simulink model "biplex_unscr_tail_plan"  (Simulink 7.6)
settings: Solver=ode45  StartTime=0.0  StopTime=10.0  RelTol=1e-3
libraries: xbsIndex_r4 x206, monroe_library x3
(part 1 of 2)
settings Model: Creator=monroe  LastModifiedBy=monroe

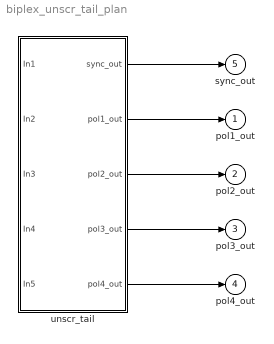
== system biplex_unscr_tail_plan ==
  unscr_tail : Subsystem  mask{FFTSize=5, input_bit_width=18, bram_latency=3, reorder_din_latency=1}
      mask prompts: FFTSize "FFT Size"; input_bit_width "Input Bit Width"; bram_latency "BRAM Latency"; reorder_din_latency "Reorder DIN Latency"
  pol1_out : Outport
  pol2_out : Outport  Port=2
  pol3_out : Outport  Port=3
  pol4_out : Outport  Port=4
  sync_out : Outport  Port=5
  wires:
  unscr_tail/5(pol4_out) -> pol4_out/1
  unscr_tail/4(pol3_out) -> pol3_out/1
  unscr_tail/3(pol2_out) -> pol2_out/1
  unscr_tail/2(pol1_out) -> pol1_out/1
  unscr_tail/1(sync_out) -> sync_out/1

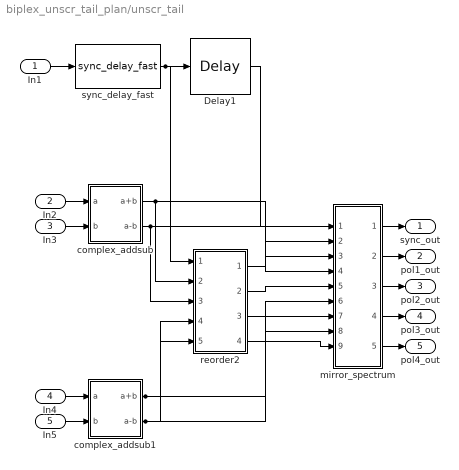
== system biplex_unscr_tail_plan/unscr_tail ==
  In1 : Inport
  In2 : Inport  Port=2
  In3 : Inport  Port=3
  In4 : Inport  Port=4
  In5 : Inport  Port=5
  Delay1 : xbsIndex_r4/Delay  en=off  latency=bram_latency + reorder_din_latency  dbl_ovrd=off  reg_retiming=off  block_type=delay
  complex_addsub : Subsystem
  complex_addsub1 : Subsystem
  mirror_spectrum : Subsystem
  reorder2 : Subsystem
  sync_delay_fast : monroe_library/sync_delay_fast  SystemSampleTime=-1  delay_len=2^(FFTSize-1) + 2
  sync_out : Outport
  pol1_out : Outport  Port=2
  pol2_out : Outport  Port=3
  pol3_out : Outport  Port=4
  pol4_out : Outport  Port=5
  wires:
  complex_addsub/2(a-b) -> reorder2/3(din1), mirror_spectrum/4(din1)
  complex_addsub/1(a+b) -> reorder2/2(din0), mirror_spectrum/2(din0)
  Delay1/1 -> mirror_spectrum/1(sync)
  reorder2/1(dout0) -> mirror_spectrum/3(reo_in0)
  reorder2/2(dout1) -> mirror_spectrum/5(reo_in1)
  reorder2/3(dout2) -> mirror_spectrum/7(reo_in2)
  reorder2/4(dout3) -> mirror_spectrum/9(reo_in3)
  complex_addsub1/2(a-b) -> mirror_spectrum/8(din3), reorder2/5(din3)
  complex_addsub1/1(a+b) -> mirror_spectrum/6(din2), reorder2/4(din2)
  sync_delay_fast/1 -> Delay1/1, reorder2/1(sync)
  In1/1 -> sync_delay_fast/1
  In2/1 -> complex_addsub/1(a)
  In3/1 -> complex_addsub/2(b)
  mirror_spectrum/1(sync_out) -> sync_out/1
  mirror_spectrum/2(dout0) -> pol1_out/1
  mirror_spectrum/3(dout1) -> pol2_out/1
  mirror_spectrum/4(dout2) -> pol3_out/1
  mirror_spectrum/5(dout3) -> pol4_out/1
  In4/1 -> complex_addsub1/1(a)
  In5/1 -> complex_addsub1/2(b)

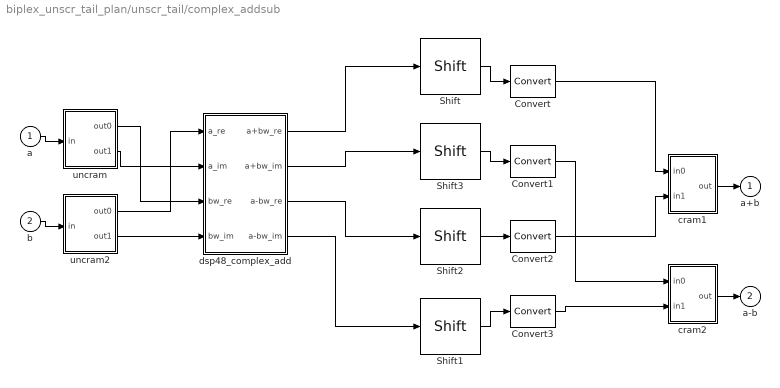
== system biplex_unscr_tail_plan/unscr_tail/complex_addsub ==
  a : Inport
  b : Inport  Port=2
  Convert{,1..3} (4 alike) : xbsIndex_r4/Convert  arith_type="Signed  (2's comp)"  n_bits=input_bit_width  bin_pt=input_bit_width-1  quantization=Truncate  overflow=Wrap  en=off  latency=0  dbl_ovrd=off  pipeline=off  block_type=convert
  Shift{,1..3} (4 alike) : xbsIndex_r4/Shift  shift_dir=Right  shift_bits=1  en=off  latency=0  precision=Full  arith_type="Signed  (2's comp)"  n_bits=8  bin_pt=2  quantization=Truncate  overflow=Wrap  dbl_ovrd=off  block_type=shift
  cram1 : Subsystem
  cram2 : Subsystem
  dsp48_complex_add : Subsystem
  uncram : Subsystem
  uncram2 : Subsystem
  a+b : Outport
  a-b : Outport  Port=2
  wires:
  a/1 -> uncram/1(in)
  b/1 -> uncram2/1(in)
  Convert/1 -> cram1/1(in0)
  Convert2/1 -> cram1/2(in1)
  cram1/1(out) -> a+b/1
  Convert1/1 -> cram2/1(in0)
  Convert3/1 -> cram2/2(in1)
  cram2/1(out) -> a-b/1
  uncram2/1(out0) -> dsp48_complex_add/1(a_re)
  uncram/2(out1) -> dsp48_complex_add/2(a_im)
  uncram/1(out0) -> dsp48_complex_add/3(bw_re)
  uncram2/2(out1) -> dsp48_complex_add/4(bw_im)
  dsp48_complex_add/1(a+bw_re) -> Shift/1
  dsp48_complex_add/2(a+bw_im) -> Shift3/1
  dsp48_complex_add/3(a-bw_re) -> Shift2/1
  dsp48_complex_add/4(a-bw_im) -> Shift1/1
  Shift1/1 -> Convert3/1
  Shift2/1 -> Convert2/1
  Shift3/1 -> Convert1/1
  Shift/1 -> Convert/1

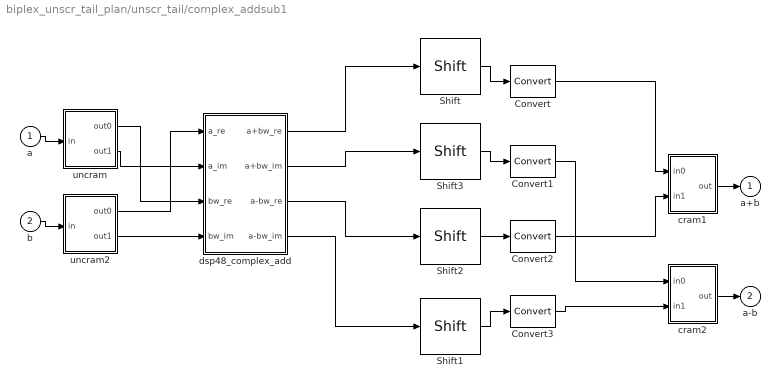
== system biplex_unscr_tail_plan/unscr_tail/complex_addsub1 ==
  a : Inport
  b : Inport  Port=2
  Convert{,1..3} (4 alike) : xbsIndex_r4/Convert  arith_type="Signed  (2's comp)"  n_bits=input_bit_width  bin_pt=input_bit_width-1  quantization=Truncate  overflow=Wrap  en=off  latency=0  dbl_ovrd=off  pipeline=off  block_type=convert
  Shift{,1..3} (4 alike) : xbsIndex_r4/Shift  shift_dir=Right  shift_bits=1  en=off  latency=0  precision=Full  arith_type="Signed  (2's comp)"  n_bits=8  bin_pt=2  quantization=Truncate  overflow=Wrap  dbl_ovrd=off  block_type=shift
  cram1 : Subsystem
  cram2 : Subsystem
  dsp48_complex_add : Subsystem
  uncram : Subsystem
  uncram2 : Subsystem
  a+b : Outport
  a-b : Outport  Port=2
  wires:
  Shift/1 -> Convert/1
  Shift3/1 -> Convert1/1
  Shift2/1 -> Convert2/1
  Shift1/1 -> Convert3/1
  dsp48_complex_add/4(a-bw_im) -> Shift1/1
  dsp48_complex_add/3(a-bw_re) -> Shift2/1
  dsp48_complex_add/2(a+bw_im) -> Shift3/1
  dsp48_complex_add/1(a+bw_re) -> Shift/1
  uncram2/2(out1) -> dsp48_complex_add/4(bw_im)
  uncram/1(out0) -> dsp48_complex_add/3(bw_re)
  uncram/2(out1) -> dsp48_complex_add/2(a_im)
  uncram2/1(out0) -> dsp48_complex_add/1(a_re)
  cram2/1(out) -> a-b/1
  Convert3/1 -> cram2/2(in1)
  Convert1/1 -> cram2/1(in0)
  cram1/1(out) -> a+b/1
  Convert2/1 -> cram1/2(in1)
  Convert/1 -> cram1/1(in0)
  b/1 -> uncram2/1(in)
  a/1 -> uncram/1(in)

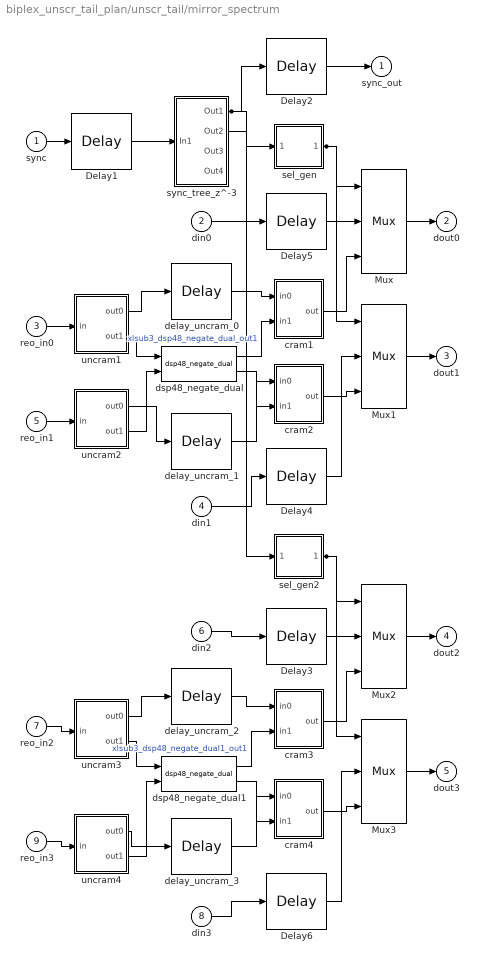
== system biplex_unscr_tail_plan/unscr_tail/mirror_spectrum ==
  sync : Inport
  din0 : Inport  Port=2
  reo_in0 : Inport  Port=3
  din1 : Inport  Port=4
  reo_in1 : Inport  Port=5
  din2 : Inport  Port=6
  reo_in2 : Inport  Port=7
  din3 : Inport  Port=8
  reo_in3 : Inport  Port=9
  Delay1 : xbsIndex_r4/Delay  en=off  latency=0  dbl_ovrd=off  reg_retiming=off  block_type=delay
  Delay2 : xbsIndex_r4/Delay  en=off  latency=1  dbl_ovrd=off  reg_retiming=off  block_type=delay
  Delay{3..6} (4 alike) : xbsIndex_r4/Delay  en=off  latency=bram_latency + 2 + reorder_din_latency  dbl_ovrd=off  reg_retiming=off  block_type=delay
  Mux{,1..3} (4 alike) : xbsIndex_r4/Mux  inputs=2  en=off  latency=0  precision=Full  arith_type="Signed  (2's comp)"  n_bits=8  bin_pt=2  quantization=Truncate  overflow=Wrap  dbl_ovrd=off  block_type=mux
  cram1 : Subsystem
  cram2 : Subsystem
  cram3 : Subsystem
  cram4 : Subsystem
  delay_uncram_{0..3} (4 alike) : xbsIndex_r4/Delay  en=off  latency=2  dbl_ovrd=off  reg_retiming=off  block_type=delay
  dsp48_negate_dual : monroe_library/dsp48_negate_dual  SystemSampleTime=-1  a_bit_width=input_bit_width  a_bin_pt=input_bit_width-1
  dsp48_negate_dual1 : monroe_library/dsp48_negate_dual  SystemSampleTime=-1  a_bit_width=input_bit_width  a_bin_pt=input_bit_width-1
  sel_gen : Subsystem
  sel_gen2 : Subsystem
  sync_tree_z^-3 : Subsystem
  uncram1 : Subsystem
  uncram2 : Subsystem
  uncram3 : Subsystem
  uncram4 : Subsystem
  sync_out : Outport
  dout0 : Outport  Port=2
  dout1 : Outport  Port=3
  dout2 : Outport  Port=4
  dout3 : Outport  Port=5
  wires:
  reo_in0/1 -> uncram1/1(in)
  reo_in1/1 -> uncram2/1(in)
  reo_in2/1 -> uncram3/1(in)
  reo_in3/1 -> uncram4/1(in)
  uncram1/1(out0) -> delay_uncram_0/1
  uncram2/1(out0) -> delay_uncram_1/1
  uncram3/1(out0) -> delay_uncram_2/1
  uncram4/1(out0) -> delay_uncram_3/1
  sync/1 -> Delay1/1
  Delay2/1 -> sync_out/1
  din2/1 -> Delay3/1
  din1/1 -> Delay4/1
  din0/1 -> Delay5/1
  din3/1 -> Delay6/1
  Delay5/1 -> Mux/2
  Mux/1 -> dout0/1
  Delay4/1 -> Mux1/2
  Mux1/1 -> dout1/1
  Delay3/1 -> Mux2/2
  Mux2/1 -> dout2/1
  Delay6/1 -> Mux3/2
  Mux3/1 -> dout3/1
  uncram1/2(out1) -> dsp48_negate_dual/1
  uncram2/2(out1) -> dsp48_negate_dual/2
  uncram3/2(out1) -> dsp48_negate_dual1/1
  uncram4/2(out1) -> dsp48_negate_dual1/2
  delay_uncram_0/1 -> cram1/1(in0)
  dsp48_negate_dual/1 -> cram1/2(in1)  "xlsub3_dsp48_negate_dual_out1"
  cram1/1(out) -> Mux/3
  delay_uncram_1/1 -> cram2/1(in0)
  dsp48_negate_dual/2 -> cram2/2(in1)
  cram2/1(out) -> Mux1/3
  delay_uncram_2/1 -> cram3/1(in0)
  dsp48_negate_dual1/1 -> cram3/2(in1)  "xlsub3_dsp48_negate_dual1_out1"
  cram3/1(out) -> Mux2/3
  delay_uncram_3/1 -> cram4/1(in0)
  dsp48_negate_dual1/2 -> cram4/2(in1)
  cram4/1(out) -> Mux3/3
  Delay1/1 -> sync_tree_z^-3/1(In1)
  sync_tree_z^-3/2(Out2) -> sel_gen2/1(sync_in)
  sync_tree_z^-3/1(Out1) -> Delay2/1, sel_gen/1(sync_in)
  sel_gen2/1(sel_out) -> Mux2/1, Mux3/1
  sel_gen/1(sel_out) -> Mux/1, Mux1/1

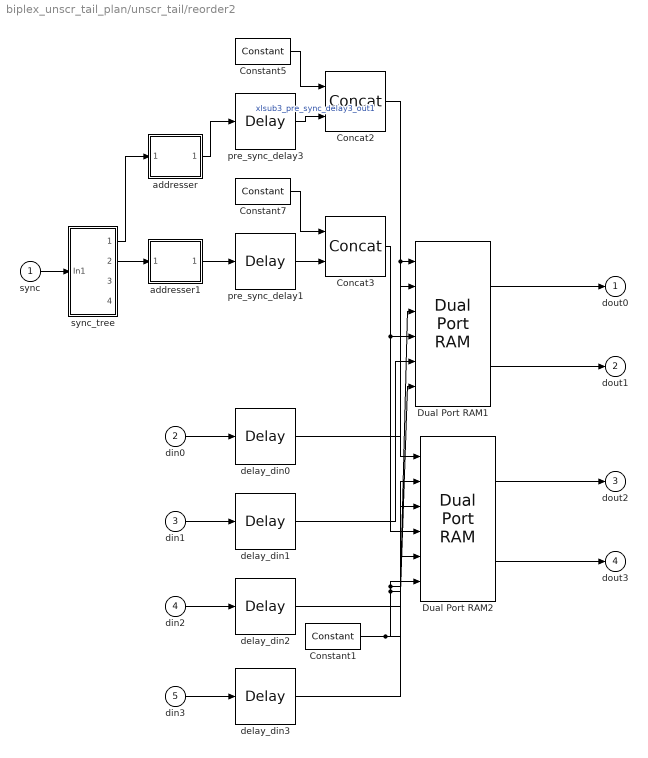
== system biplex_unscr_tail_plan/unscr_tail/reorder2 ==
  sync : Inport
  din0 : Inport  Port=2
  din1 : Inport  Port=3
  din2 : Inport  Port=4
  din3 : Inport  Port=5
  Concat2 : xbsIndex_r4/Concat  num_inputs=2  dbl_ovrd=off  block_type=concat
  Concat3 : xbsIndex_r4/Concat  num_inputs=2  dbl_ovrd=off  block_type=concat
  Constant1 : xbsIndex_r4/Constant  arith_type=Boolean  const=1  n_bits=1  bin_pt=0  explicit_period=on  period=1  equ=P=C  opselect=C  inp2=PCIN>>17  opr=+  inp1=P  carry=CIN  dbl_ovrd=off  block_type=constant
  Constant5 : xbsIndex_r4/Constant  arith_type=Boolean  const=1  n_bits=1  bin_pt=0  explicit_period=on  period=1  equ=P=C  opselect=C  inp2=PCIN>>17  opr=+  inp1=P  carry=CIN  dbl_ovrd=off  block_type=constant
  Constant7 : xbsIndex_r4/Constant  arith_type=Boolean  const=0  n_bits=1  bin_pt=0  explicit_period=on  period=1  equ=P=C  opselect=C  inp2=PCIN>>17  opr=+  inp1=P  carry=CIN  dbl_ovrd=off  block_type=constant
  Dual Port RAM1 : xbsIndex_r4/Dual Port RAM  depth=2^FFTSize  initVector=sin(pi*(0:15)/16)  distributed_mem=Block RAM  init_a=0  init_b=0  rst_a=off  rst_b=off  en_a=off  en_b=off  latency=bram_latency  write_mode_A=Read Before Write  write_mode_B=Read Before Write  dbl_ovrd=off  optimize=Area  use_rpm=on  block_type=dpram
  Dual Port RAM2 : xbsIndex_r4/Dual Port RAM  depth=2^FFTSize  initVector=sin(pi*(0:15)/16)  distributed_mem=Block RAM  init_a=0  init_b=0  rst_a=off  rst_b=off  en_a=off  en_b=off  latency=bram_latency  write_mode_A=Read Before Write  write_mode_B=Read Before Write  dbl_ovrd=off  optimize=Area  use_rpm=on  block_type=dpram
  addresser : Subsystem
  addresser1 : Subsystem
  delay_din{0..3} (4 alike) : xbsIndex_r4/Delay  en=off  latency=reorder_din_latency  dbl_ovrd=off  reg_retiming=off  block_type=delay
  pre_sync_delay1 : xbsIndex_r4/Delay  en=off  latency=reorder_din_latency  dbl_ovrd=off  reg_retiming=off  block_type=delay
  pre_sync_delay3 : xbsIndex_r4/Delay  en=off  latency=reorder_din_latency  dbl_ovrd=off  reg_retiming=off  block_type=delay
  sync_tree : Subsystem
  dout0 : Outport
  dout1 : Outport  Port=2
  dout2 : Outport  Port=3
  dout3 : Outport  Port=4
  wires:
  Constant5/1 -> Concat2/1
  Constant7/1 -> Concat3/1
  Concat2/1 -> Dual Port RAM1/1, Dual Port RAM2/1
  Concat3/1 -> Dual Port RAM1/4, Dual Port RAM2/4
  Dual Port RAM1/2 -> dout1/1
  Dual Port RAM1/1 -> dout0/1
  din0/1 -> delay_din0/1
  din1/1 -> delay_din1/1
  din2/1 -> delay_din2/1
  din3/1 -> delay_din3/1
  pre_sync_delay1/1 -> Concat3/2
  pre_sync_delay3/1 -> Concat2/2  "xlsub3_pre_sync_delay3_out1"
  addresser/1(addr_out) -> pre_sync_delay3/1
  addresser1/1(addr_out) -> pre_sync_delay1/1
  sync/1 -> sync_tree/1(In1)
  sync_tree/2(Out2) -> addresser1/1(sync_in)
  sync_tree/1(Out1) -> addresser/1(sync_in)
  Dual Port RAM2/2 -> dout3/1
  Dual Port RAM2/1 -> dout2/1
  Constant1/1 -> Dual Port RAM1/6, Dual Port RAM1/3, Dual Port RAM2/6, Dual Port RAM2/3
  delay_din0/1 -> Dual Port RAM1/2
  delay_din1/1 -> Dual Port RAM1/5
  delay_din2/1 -> Dual Port RAM2/2
  delay_din3/1 -> Dual Port RAM2/5

== system biplex_unscr_tail_plan/unscr_tail/complex_addsub/cram1 ==
  in0 : Inport
  in1 : Inport  Port=2
  Concat5 : xbsIndex_r4/Concat  num_inputs=2  dbl_ovrd=off  block_type=concat
  Reinterpret23 : xbsIndex_r4/Reinterpret  force_arith_type=on  arith_type=Unsigned  force_bin_pt=on  bin_pt=0  block_type=reinterpret
      settings: infoedit="Changes signal type without altering the binary representation.   You can changed the signal between signed and unsigned, and relocate the binary point.<br><br>Hardware notes: In hardware this block costs nothing.<br><br>Example:  Suppose the input is 6 bits wide, signed, with 2 fractional bits, and the output is forced to unsigned with 0 fractional bits.  Then an input of -2.0 (1110.00 in binary 2's complement) becomes an output of 56 (111000 in binary)."
  Reinterpret24 : xbsIndex_r4/Reinterpret  force_arith_type=on  arith_type=Unsigned  force_bin_pt=on  bin_pt=0  block_type=reinterpret
      settings: infoedit="Changes signal type without altering the binary representation.   You can changed the signal between signed and unsigned, and relocate the binary point.<br><br>Hardware notes: In hardware this block costs nothing.<br><br>Example:  Suppose the input is 6 bits wide, signed, with 2 fractional bits, and the output is forced to unsigned with 0 fractional bits.  Then an input of -2.0 (1110.00 in binary 2's complement) becomes an output of 56 (111000 in binary)."
  out : Outport
  wires:
  Reinterpret24/1 -> Concat5/2
  in1/1 -> Reinterpret24/1
  Reinterpret23/1 -> Concat5/1
  in0/1 -> Reinterpret23/1
  Concat5/1 -> out/1

== system biplex_unscr_tail_plan/unscr_tail/complex_addsub/cram2 ==
  in0 : Inport
  in1 : Inport  Port=2
  Concat5 : xbsIndex_r4/Concat  num_inputs=2  dbl_ovrd=off  block_type=concat
  Reinterpret23 : xbsIndex_r4/Reinterpret  force_arith_type=on  arith_type=Unsigned  force_bin_pt=on  bin_pt=0  block_type=reinterpret
      settings: infoedit="Changes signal type without altering the binary representation.   You can changed the signal between signed and unsigned, and relocate the binary point.<br><br>Hardware notes: In hardware this block costs nothing.<br><br>Example:  Suppose the input is 6 bits wide, signed, with 2 fractional bits, and the output is forced to unsigned with 0 fractional bits.  Then an input of -2.0 (1110.00 in binary 2's complement) becomes an output of 56 (111000 in binary)."
  Reinterpret24 : xbsIndex_r4/Reinterpret  force_arith_type=on  arith_type=Unsigned  force_bin_pt=on  bin_pt=0  block_type=reinterpret
      settings: infoedit="Changes signal type without altering the binary representation.   You can changed the signal between signed and unsigned, and relocate the binary point.<br><br>Hardware notes: In hardware this block costs nothing.<br><br>Example:  Suppose the input is 6 bits wide, signed, with 2 fractional bits, and the output is forced to unsigned with 0 fractional bits.  Then an input of -2.0 (1110.00 in binary 2's complement) becomes an output of 56 (111000 in binary)."
  out : Outport
  wires:
  Concat5/1 -> out/1
  in0/1 -> Reinterpret23/1
  Reinterpret23/1 -> Concat5/1
  in1/1 -> Reinterpret24/1
  Reinterpret24/1 -> Concat5/2

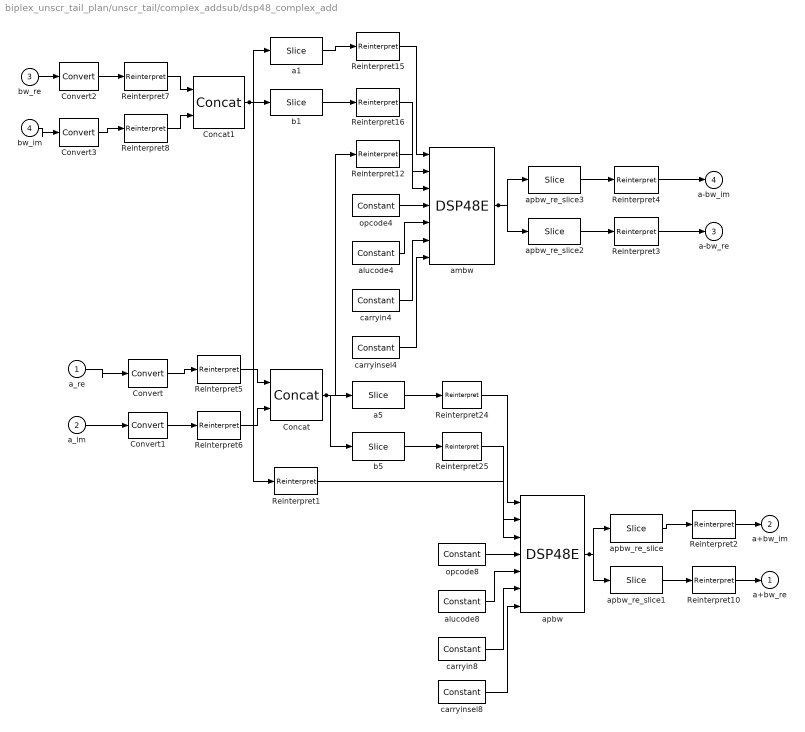
== system biplex_unscr_tail_plan/unscr_tail/complex_addsub/dsp48_complex_add ==
  a_re : Inport
  a_im : Inport  Port=2
  bw_re : Inport  Port=3
  bw_im : Inport  Port=4
  Concat : xbsIndex_r4/Concat  num_inputs=2  dbl_ovrd=off  block_type=concat
  Concat1 : xbsIndex_r4/Concat  num_inputs=2  dbl_ovrd=off  block_type=concat
  Convert{,1..3} (4 alike) : xbsIndex_r4/Convert  arith_type="Signed  (2's comp)"  n_bits=24  bin_pt=22  quantization=Truncate  overflow=Wrap  en=off  latency=0  dbl_ovrd=off  pipeline=off  block_type=convert
  Reinterpret{1,12,15..16,24..25} (6 alike) : xbsIndex_r4/Reinterpret  force_arith_type=on  arith_type="Signed  (2's comp)"  force_bin_pt=off  bin_pt=0  block_type=reinterpret
      settings: infoedit="Changes signal type without altering the binary representation.   You can changed the signal between signed and unsigned, and relocate the binary point.<br><br>Hardware notes: In hardware this block costs nothing.<br><br>Example:  Suppose the input is 6 bits wide, signed, with 2 fractional bits, and the output is forced to unsigned with 0 fractional bits.  Then an input of -2.0 (1110.00 in binary 2's complement) becomes an output of 56 (111000 in binary)."
  Reinterpret{2..4,10} (4 alike) : xbsIndex_r4/Reinterpret  force_arith_type=on  arith_type="Signed  (2's comp)"  force_bin_pt=on  bin_pt=22  block_type=reinterpret
      settings: infoedit="Changes signal type without altering the binary representation.   You can changed the signal between signed and unsigned, and relocate the binary point.<br><br>Hardware notes: In hardware this block costs nothing.<br><br>Example:  Suppose the input is 6 bits wide, signed, with 2 fractional bits, and the output is forced to unsigned with 0 fractional bits.  Then an input of -2.0 (1110.00 in binary 2's complement) becomes an output of 56 (111000 in binary)."
  Reinterpret{5..8} (4 alike) : xbsIndex_r4/Reinterpret  force_arith_type=on  arith_type=Unsigned  force_bin_pt=on  bin_pt=0  block_type=reinterpret
      settings: infoedit="Changes signal type without altering the binary representation.   You can changed the signal between signed and unsigned, and relocate the binary point.<br><br>Hardware notes: In hardware this block costs nothing.<br><br>Example:  Suppose the input is 6 bits wide, signed, with 2 fractional bits, and the output is forced to unsigned with 0 fractional bits.  Then an input of -2.0 (1110.00 in binary 2's complement) becomes an output of 56 (111000 in binary)."
  a1 : xbsIndex_r4/Slice  nbits=30  boolean_output=off  mode=Upper Bit Location + Width  bit1=0  base1=MSB of Input  bit0=18  base0=LSB of Input  dbl_ovrd=off  block_type=slice
  a5 : xbsIndex_r4/Slice  nbits=30  boolean_output=off  mode=Upper Bit Location + Width  bit1=0  base1=MSB of Input  bit0=18  base0=LSB of Input  dbl_ovrd=off  block_type=slice
  alucode4 : xbsIndex_r4/Constant  arith_type=Unsigned  const=3  n_bits=4  bin_pt=0  explicit_period=on  period=1  equ=P=C  opselect=C  inp2=PCIN>>17  opr=+  inp1=P  carry=CIN  dbl_ovrd=off  block_type=constant
  alucode8 : xbsIndex_r4/Constant  arith_type=Unsigned  const=0  n_bits=4  bin_pt=0  explicit_period=on  period=1  equ=P=C  opselect=C  inp2=PCIN>>17  opr=+  inp1=P  carry=CIN  dbl_ovrd=off  block_type=constant
  ambw : xbsIndex_r4/DSP48E  use_a=Direct from A Port  use_b=Direct from B Port  reset_preg=off  pattern_from_creg=off  pattern='000000000000'  mask_from_creg=off  pattern_mask='3FFFFFFFFFFF'  sel_rounding_mask=Select mask  use_op=off  use_creg=on  rst_all=off  en_all=off  use_pcin=off  use_carrycascin=off  use_multsignin=off  use_carryout=off  use_patterndetect=off  use_patternbdetect=off  use_overflow=off  use_underflow=off  use_acout=off  use_bcout=off  use_pcout=off  use_multsignout=off  use_carrycascout=off  pipeline_a=1  pipeline_b=1  pipeline_acout=1  pipeline_bcout=1  pipeline_c=on  pipeline_p=on  pipeline_mult=on  pipeline_opmode=on  pipeline_alumode=on  pipeline_carryin=on  pipeline_carryinsel=on  rst_a=off  rst_b=off  rst_c=off  rst_mult=off  rst_p=off  rst_carry_in=off  rst_alumode=off  rst_ctrl=off  en_a1=off  en_a2=off  en_b1=off  en_b2=off  en_c=off  en_mult=off  en_p=off  en_carry_in=off  en_alumode=off  en_multcarryin=off  en_ctrl=off  use_synth_model=off  addsub_mode=TWO24  xl_useadderonly=off  block_type=dsp48e
  apbw : xbsIndex_r4/DSP48E  use_a=Direct from A Port  use_b=Direct from B Port  reset_preg=off  pattern_from_creg=off  pattern='000000000000'  mask_from_creg=off  pattern_mask='3FFFFFFFFFFF'  sel_rounding_mask=Select mask  use_op=off  use_creg=on  rst_all=off  en_all=off  use_pcin=off  use_carrycascin=off  use_multsignin=off  use_carryout=off  use_patterndetect=off  use_patternbdetect=off  use_overflow=off  use_underflow=off  use_acout=off  use_bcout=off  use_pcout=off  use_multsignout=off  use_carrycascout=off  pipeline_a=1  pipeline_b=1  pipeline_acout=1  pipeline_bcout=1  pipeline_c=on  pipeline_p=on  pipeline_mult=on  pipeline_opmode=on  pipeline_alumode=on  pipeline_carryin=on  pipeline_carryinsel=on  rst_a=off  rst_b=off  rst_c=off  rst_mult=off  rst_p=off  rst_carry_in=off  rst_alumode=off  rst_ctrl=off  en_a1=off  en_a2=off  en_b1=off  en_b2=off  en_c=off  en_mult=off  en_p=off  en_carry_in=off  en_alumode=off  en_multcarryin=off  en_ctrl=off  use_synth_model=off  addsub_mode=TWO24  xl_useadderonly=off  block_type=dsp48e
  apbw_re_slice : xbsIndex_r4/Slice  nbits=24  boolean_output=off  mode=Lower Bit Location + Width  bit1=0  base1=MSB of Input  bit0=0  base0=LSB of Input  dbl_ovrd=off  block_type=slice
  apbw_re_slice1 : xbsIndex_r4/Slice  nbits=24  boolean_output=off  mode=Upper Bit Location + Width  bit1=0  base1=MSB of Input  bit0=24  base0=LSB of Input  dbl_ovrd=off  block_type=slice
  apbw_re_slice2 : xbsIndex_r4/Slice  nbits=24  boolean_output=off  mode=Upper Bit Location + Width  bit1=0  base1=MSB of Input  bit0=24  base0=LSB of Input  dbl_ovrd=off  block_type=slice
  apbw_re_slice3 : xbsIndex_r4/Slice  nbits=24  boolean_output=off  mode=Lower Bit Location + Width  bit1=0  base1=MSB of Input  bit0=0  base0=LSB of Input  dbl_ovrd=off  block_type=slice
  b1 : xbsIndex_r4/Slice  nbits=18  boolean_output=off  mode=Lower Bit Location + Width  bit1=0  base1=MSB of Input  bit0=0  base0=LSB of Input  dbl_ovrd=off  block_type=slice
  b5 : xbsIndex_r4/Slice  nbits=18  boolean_output=off  mode=Lower Bit Location + Width  bit1=0  base1=MSB of Input  bit0=0  base0=LSB of Input  dbl_ovrd=off  block_type=slice
  carryin4 : xbsIndex_r4/Constant  arith_type=Unsigned  const=0  n_bits=1  bin_pt=0  explicit_period=on  period=1  equ=P=C  opselect=C  inp2=PCIN>>17  opr=+  inp1=P  carry=CIN  dbl_ovrd=off  block_type=constant
  carryin8 : xbsIndex_r4/Constant  arith_type=Unsigned  const=0  n_bits=1  bin_pt=0  explicit_period=on  period=1  equ=P=C  opselect=C  inp2=PCIN>>17  opr=+  inp1=P  carry=CIN  dbl_ovrd=off  block_type=constant
  carryinsel4 : xbsIndex_r4/Constant  arith_type=Unsigned  const=0  n_bits=3  bin_pt=0  explicit_period=on  period=1  equ=P=C  opselect=C  inp2=PCIN>>17  opr=+  inp1=P  carry=CIN  dbl_ovrd=off  block_type=constant
  carryinsel8 : xbsIndex_r4/Constant  arith_type=Unsigned  const=0  n_bits=3  bin_pt=0  explicit_period=on  period=1  equ=P=C  opselect=C  inp2=PCIN>>17  opr=+  inp1=P  carry=CIN  dbl_ovrd=off  block_type=constant
  opcode4 : xbsIndex_r4/Constant  arith_type=Unsigned  const=51  n_bits=7  bin_pt=0  explicit_period=on  period=1  equ=P=C  opselect=C  inp2=PCIN>>17  opr=+  inp1=P  carry=CIN  dbl_ovrd=off  block_type=constant
  opcode8 : xbsIndex_r4/Constant  arith_type=Unsigned  const=15  n_bits=7  bin_pt=0  explicit_period=on  period=1  equ=P=C  opselect=C  inp2=PCIN>>17  opr=+  inp1=P  carry=CIN  dbl_ovrd=off  block_type=constant
  a+bw_re : Outport
  a+bw_im : Outport  Port=2
  a-bw_re : Outport  Port=3
  a-bw_im : Outport  Port=4
  wires:
  a_re/1 -> Convert/1
  a_im/1 -> Convert1/1
  bw_re/1 -> Convert2/1
  bw_im/1 -> Convert3/1
  Reinterpret10/1 -> a+bw_re/1
  Reinterpret2/1 -> a+bw_im/1
  Reinterpret3/1 -> a-bw_re/1
  Reinterpret4/1 -> a-bw_im/1
  Convert/1 -> Reinterpret5/1
  Reinterpret5/1 -> Concat/1
  Convert1/1 -> Reinterpret6/1
  Reinterpret6/1 -> Concat/2
  Convert2/1 -> Reinterpret7/1
  Reinterpret7/1 -> Concat1/1
  Convert3/1 -> Reinterpret8/1
  Reinterpret8/1 -> Concat1/2
  a1/1 -> Reinterpret15/1
  a5/1 -> Reinterpret24/1
  Reinterpret15/1 -> ambw/1
  Reinterpret16/1 -> ambw/2
  Reinterpret12/1 -> ambw/3
  alucode4/1 -> ambw/5
  Reinterpret24/1 -> apbw/1
  Reinterpret25/1 -> apbw/2
  Reinterpret1/1 -> apbw/3
  alucode8/1 -> apbw/5
  apbw_re_slice/1 -> Reinterpret2/1
  apbw_re_slice1/1 -> Reinterpret10/1
  apbw_re_slice2/1 -> Reinterpret3/1
  apbw_re_slice3/1 -> Reinterpret4/1
  b1/1 -> Reinterpret16/1
  b5/1 -> Reinterpret25/1
  carryin4/1 -> ambw/6
  carryin8/1 -> apbw/6
  carryinsel4/1 -> ambw/7
  carryinsel8/1 -> apbw/7
  opcode4/1 -> ambw/4
  opcode8/1 -> apbw/4
  ambw/1 -> apbw_re_slice2/1, apbw_re_slice3/1
  apbw/1 -> apbw_re_slice/1, apbw_re_slice1/1
  Concat/1 -> Reinterpret12/1, a5/1, b5/1
  Concat1/1 -> Reinterpret1/1, a1/1, b1/1

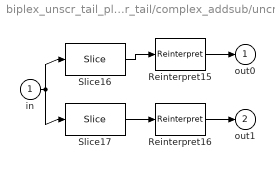
== system biplex_unscr_tail_plan/unscr_tail/complex_addsub/uncram ==
  in : Inport
  Reinterpret15 : xbsIndex_r4/Reinterpret  force_arith_type=on  arith_type="Signed  (2's comp)"  force_bin_pt=on  bin_pt=input_bit_width-1  block_type=reinterpret
      settings: infoedit="Changes signal type without altering the binary representation.   You can changed the signal between signed and unsigned, and relocate the binary point.<br><br>Hardware notes: In hardware this block costs nothing.<br><br>Example:  Suppose the input is 6 bits wide, signed, with 2 fractional bits, and the output is forced to unsigned with 0 fractional bits.  Then an input of -2.0 (1110.00 in binary 2's complement) becomes an output of 56 (111000 in binary)."
  Reinterpret16 : xbsIndex_r4/Reinterpret  force_arith_type=on  arith_type="Signed  (2's comp)"  force_bin_pt=on  bin_pt=input_bit_width-1  block_type=reinterpret
      settings: infoedit="Changes signal type without altering the binary representation.   You can changed the signal between signed and unsigned, and relocate the binary point.<br><br>Hardware notes: In hardware this block costs nothing.<br><br>Example:  Suppose the input is 6 bits wide, signed, with 2 fractional bits, and the output is forced to unsigned with 0 fractional bits.  Then an input of -2.0 (1110.00 in binary 2's complement) becomes an output of 56 (111000 in binary)."
  Slice16 : xbsIndex_r4/Slice  nbits=input_bit_width  boolean_output=off  mode=Upper Bit Location + Width  bit1=-0  base1=MSB of Input  bit0=0  base0=MSB of Input  dbl_ovrd=off  block_type=slice
  Slice17 : xbsIndex_r4/Slice  nbits=input_bit_width  boolean_output=off  mode=Upper Bit Location + Width  bit1=-1* input_bit_width  base1=MSB of Input  bit0=0  base0=MSB of Input  dbl_ovrd=off  block_type=slice
  out0 : Outport
  out1 : Outport  Port=2
  wires:
  in/1 -> Slice17/1, Slice16/1
  Reinterpret16/1 -> out1/1
  Slice17/1 -> Reinterpret16/1
  Reinterpret15/1 -> out0/1
  Slice16/1 -> Reinterpret15/1

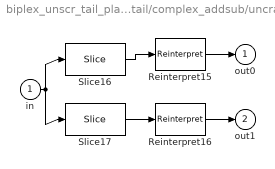
== system biplex_unscr_tail_plan/unscr_tail/complex_addsub/uncram2 ==
  in : Inport
  Reinterpret15 : xbsIndex_r4/Reinterpret  force_arith_type=on  arith_type="Signed  (2's comp)"  force_bin_pt=on  bin_pt=input_bit_width-1  block_type=reinterpret
      settings: infoedit="Changes signal type without altering the binary representation.   You can changed the signal between signed and unsigned, and relocate the binary point.<br><br>Hardware notes: In hardware this block costs nothing.<br><br>Example:  Suppose the input is 6 bits wide, signed, with 2 fractional bits, and the output is forced to unsigned with 0 fractional bits.  Then an input of -2.0 (1110.00 in binary 2's complement) becomes an output of 56 (111000 in binary)."
  Reinterpret16 : xbsIndex_r4/Reinterpret  force_arith_type=on  arith_type="Signed  (2's comp)"  force_bin_pt=on  bin_pt=input_bit_width-1  block_type=reinterpret
      settings: infoedit="Changes signal type without altering the binary representation.   You can changed the signal between signed and unsigned, and relocate the binary point.<br><br>Hardware notes: In hardware this block costs nothing.<br><br>Example:  Suppose the input is 6 bits wide, signed, with 2 fractional bits, and the output is forced to unsigned with 0 fractional bits.  Then an input of -2.0 (1110.00 in binary 2's complement) becomes an output of 56 (111000 in binary)."
  Slice16 : xbsIndex_r4/Slice  nbits=input_bit_width  boolean_output=off  mode=Upper Bit Location + Width  bit1=-0  base1=MSB of Input  bit0=0  base0=MSB of Input  dbl_ovrd=off  block_type=slice
  Slice17 : xbsIndex_r4/Slice  nbits=input_bit_width  boolean_output=off  mode=Upper Bit Location + Width  bit1=-1* input_bit_width  base1=MSB of Input  bit0=0  base0=MSB of Input  dbl_ovrd=off  block_type=slice
  out0 : Outport
  out1 : Outport  Port=2
  wires:
  Slice16/1 -> Reinterpret15/1
  Reinterpret15/1 -> out0/1
  Slice17/1 -> Reinterpret16/1
  Reinterpret16/1 -> out1/1
  in/1 -> Slice16/1, Slice17/1

== system biplex_unscr_tail_plan/unscr_tail/complex_addsub1/cram1 ==
  in0 : Inport
  in1 : Inport  Port=2
  Concat5 : xbsIndex_r4/Concat  num_inputs=2  dbl_ovrd=off  block_type=concat
  Reinterpret23 : xbsIndex_r4/Reinterpret  force_arith_type=on  arith_type=Unsigned  force_bin_pt=on  bin_pt=0  block_type=reinterpret
      settings: infoedit="Changes signal type without altering the binary representation.   You can changed the signal between signed and unsigned, and relocate the binary point.<br><br>Hardware notes: In hardware this block costs nothing.<br><br>Example:  Suppose the input is 6 bits wide, signed, with 2 fractional bits, and the output is forced to unsigned with 0 fractional bits.  Then an input of -2.0 (1110.00 in binary 2's complement) becomes an output of 56 (111000 in binary)."
  Reinterpret24 : xbsIndex_r4/Reinterpret  force_arith_type=on  arith_type=Unsigned  force_bin_pt=on  bin_pt=0  block_type=reinterpret
      settings: infoedit="Changes signal type without altering the binary representation.   You can changed the signal between signed and unsigned, and relocate the binary point.<br><br>Hardware notes: In hardware this block costs nothing.<br><br>Example:  Suppose the input is 6 bits wide, signed, with 2 fractional bits, and the output is forced to unsigned with 0 fractional bits.  Then an input of -2.0 (1110.00 in binary 2's complement) becomes an output of 56 (111000 in binary)."
  out : Outport
  wires:
  Concat5/1 -> out/1
  in0/1 -> Reinterpret23/1
  Reinterpret23/1 -> Concat5/1
  in1/1 -> Reinterpret24/1
  Reinterpret24/1 -> Concat5/2

== system biplex_unscr_tail_plan/unscr_tail/complex_addsub1/cram2 ==
  in0 : Inport
  in1 : Inport  Port=2
  Concat5 : xbsIndex_r4/Concat  num_inputs=2  dbl_ovrd=off  block_type=concat
  Reinterpret23 : xbsIndex_r4/Reinterpret  force_arith_type=on  arith_type=Unsigned  force_bin_pt=on  bin_pt=0  block_type=reinterpret
      settings: infoedit="Changes signal type without altering the binary representation.   You can changed the signal between signed and unsigned, and relocate the binary point.<br><br>Hardware notes: In hardware this block costs nothing.<br><br>Example:  Suppose the input is 6 bits wide, signed, with 2 fractional bits, and the output is forced to unsigned with 0 fractional bits.  Then an input of -2.0 (1110.00 in binary 2's complement) becomes an output of 56 (111000 in binary)."
  Reinterpret24 : xbsIndex_r4/Reinterpret  force_arith_type=on  arith_type=Unsigned  force_bin_pt=on  bin_pt=0  block_type=reinterpret
      settings: infoedit="Changes signal type without altering the binary representation.   You can changed the signal between signed and unsigned, and relocate the binary point.<br><br>Hardware notes: In hardware this block costs nothing.<br><br>Example:  Suppose the input is 6 bits wide, signed, with 2 fractional bits, and the output is forced to unsigned with 0 fractional bits.  Then an input of -2.0 (1110.00 in binary 2's complement) becomes an output of 56 (111000 in binary)."
  out : Outport
  wires:
  Reinterpret24/1 -> Concat5/2
  in1/1 -> Reinterpret24/1
  Reinterpret23/1 -> Concat5/1
  in0/1 -> Reinterpret23/1
  Concat5/1 -> out/1

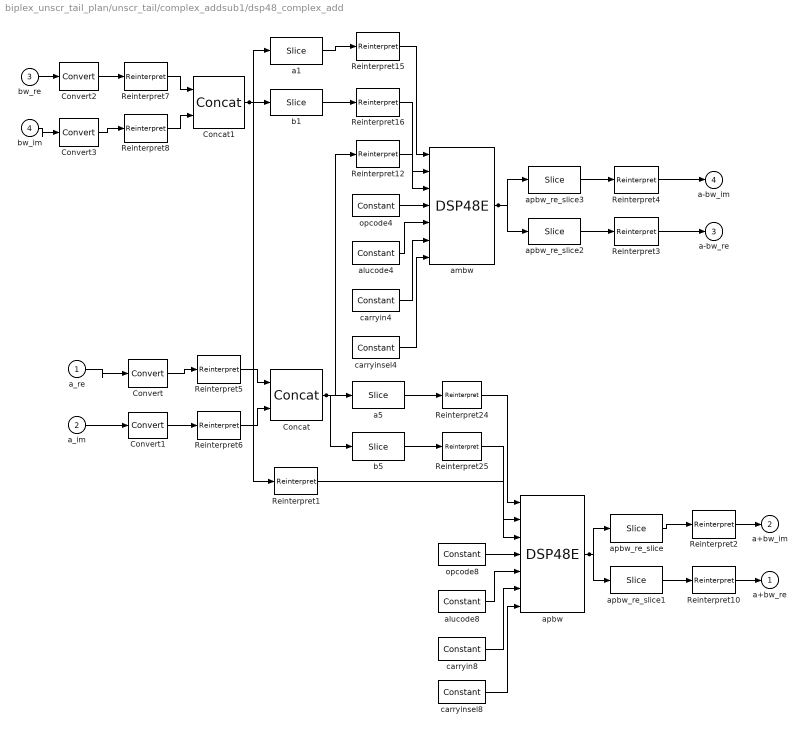
== system biplex_unscr_tail_plan/unscr_tail/complex_addsub1/dsp48_complex_add ==
  a_re : Inport
  a_im : Inport  Port=2
  bw_re : Inport  Port=3
  bw_im : Inport  Port=4
  Concat : xbsIndex_r4/Concat  num_inputs=2  dbl_ovrd=off  block_type=concat
  Concat1 : xbsIndex_r4/Concat  num_inputs=2  dbl_ovrd=off  block_type=concat
  Convert{,1..3} (4 alike) : xbsIndex_r4/Convert  arith_type="Signed  (2's comp)"  n_bits=24  bin_pt=22  quantization=Truncate  overflow=Wrap  en=off  latency=0  dbl_ovrd=off  pipeline=off  block_type=convert
  Reinterpret{1,12,15..16,24..25} (6 alike) : xbsIndex_r4/Reinterpret  force_arith_type=on  arith_type="Signed  (2's comp)"  force_bin_pt=off  bin_pt=0  block_type=reinterpret
      settings: infoedit="Changes signal type without altering the binary representation.   You can changed the signal between signed and unsigned, and relocate the binary point.<br><br>Hardware notes: In hardware this block costs nothing.<br><br>Example:  Suppose the input is 6 bits wide, signed, with 2 fractional bits, and the output is forced to unsigned with 0 fractional bits.  Then an input of -2.0 (1110.00 in binary 2's complement) becomes an output of 56 (111000 in binary)."
  Reinterpret{2..4,10} (4 alike) : xbsIndex_r4/Reinterpret  force_arith_type=on  arith_type="Signed  (2's comp)"  force_bin_pt=on  bin_pt=22  block_type=reinterpret
      settings: infoedit="Changes signal type without altering the binary representation.   You can changed the signal between signed and unsigned, and relocate the binary point.<br><br>Hardware notes: In hardware this block costs nothing.<br><br>Example:  Suppose the input is 6 bits wide, signed, with 2 fractional bits, and the output is forced to unsigned with 0 fractional bits.  Then an input of -2.0 (1110.00 in binary 2's complement) becomes an output of 56 (111000 in binary)."
  Reinterpret{5..8} (4 alike) : xbsIndex_r4/Reinterpret  force_arith_type=on  arith_type=Unsigned  force_bin_pt=on  bin_pt=0  block_type=reinterpret
      settings: infoedit="Changes signal type without altering the binary representation.   You can changed the signal between signed and unsigned, and relocate the binary point.<br><br>Hardware notes: In hardware this block costs nothing.<br><br>Example:  Suppose the input is 6 bits wide, signed, with 2 fractional bits, and the output is forced to unsigned with 0 fractional bits.  Then an input of -2.0 (1110.00 in binary 2's complement) becomes an output of 56 (111000 in binary)."
  a1 : xbsIndex_r4/Slice  nbits=30  boolean_output=off  mode=Upper Bit Location + Width  bit1=0  base1=MSB of Input  bit0=18  base0=LSB of Input  dbl_ovrd=off  block_type=slice
  a5 : xbsIndex_r4/Slice  nbits=30  boolean_output=off  mode=Upper Bit Location + Width  bit1=0  base1=MSB of Input  bit0=18  base0=LSB of Input  dbl_ovrd=off  block_type=slice
  alucode4 : xbsIndex_r4/Constant  arith_type=Unsigned  const=3  n_bits=4  bin_pt=0  explicit_period=on  period=1  equ=P=C  opselect=C  inp2=PCIN>>17  opr=+  inp1=P  carry=CIN  dbl_ovrd=off  block_type=constant
  alucode8 : xbsIndex_r4/Constant  arith_type=Unsigned  const=0  n_bits=4  bin_pt=0  explicit_period=on  period=1  equ=P=C  opselect=C  inp2=PCIN>>17  opr=+  inp1=P  carry=CIN  dbl_ovrd=off  block_type=constant
  ambw : xbsIndex_r4/DSP48E  use_a=Direct from A Port  use_b=Direct from B Port  reset_preg=off  pattern_from_creg=off  pattern='000000000000'  mask_from_creg=off  pattern_mask='3FFFFFFFFFFF'  sel_rounding_mask=Select mask  use_op=off  use_creg=on  rst_all=off  en_all=off  use_pcin=off  use_carrycascin=off  use_multsignin=off  use_carryout=off  use_patterndetect=off  use_patternbdetect=off  use_overflow=off  use_underflow=off  use_acout=off  use_bcout=off  use_pcout=off  use_multsignout=off  use_carrycascout=off  pipeline_a=1  pipeline_b=1  pipeline_acout=1  pipeline_bcout=1  pipeline_c=on  pipeline_p=on  pipeline_mult=on  pipeline_opmode=on  pipeline_alumode=on  pipeline_carryin=on  pipeline_carryinsel=on  rst_a=off  rst_b=off  rst_c=off  rst_mult=off  rst_p=off  rst_carry_in=off  rst_alumode=off  rst_ctrl=off  en_a1=off  en_a2=off  en_b1=off  en_b2=off  en_c=off  en_mult=off  en_p=off  en_carry_in=off  en_alumode=off  en_multcarryin=off  en_ctrl=off  use_synth_model=off  addsub_mode=TWO24  xl_useadderonly=off  block_type=dsp48e
  apbw : xbsIndex_r4/DSP48E  use_a=Direct from A Port  use_b=Direct from B Port  reset_preg=off  pattern_from_creg=off  pattern='000000000000'  mask_from_creg=off  pattern_mask='3FFFFFFFFFFF'  sel_rounding_mask=Select mask  use_op=off  use_creg=on  rst_all=off  en_all=off  use_pcin=off  use_carrycascin=off  use_multsignin=off  use_carryout=off  use_patterndetect=off  use_patternbdetect=off  use_overflow=off  use_underflow=off  use_acout=off  use_bcout=off  use_pcout=off  use_multsignout=off  use_carrycascout=off  pipeline_a=1  pipeline_b=1  pipeline_acout=1  pipeline_bcout=1  pipeline_c=on  pipeline_p=on  pipeline_mult=on  pipeline_opmode=on  pipeline_alumode=on  pipeline_carryin=on  pipeline_carryinsel=on  rst_a=off  rst_b=off  rst_c=off  rst_mult=off  rst_p=off  rst_carry_in=off  rst_alumode=off  rst_ctrl=off  en_a1=off  en_a2=off  en_b1=off  en_b2=off  en_c=off  en_mult=off  en_p=off  en_carry_in=off  en_alumode=off  en_multcarryin=off  en_ctrl=off  use_synth_model=off  addsub_mode=TWO24  xl_useadderonly=off  block_type=dsp48e
  apbw_re_slice : xbsIndex_r4/Slice  nbits=24  boolean_output=off  mode=Lower Bit Location + Width  bit1=0  base1=MSB of Input  bit0=0  base0=LSB of Input  dbl_ovrd=off  block_type=slice
  apbw_re_slice1 : xbsIndex_r4/Slice  nbits=24  boolean_output=off  mode=Upper Bit Location + Width  bit1=0  base1=MSB of Input  bit0=24  base0=LSB of Input  dbl_ovrd=off  block_type=slice
  apbw_re_slice2 : xbsIndex_r4/Slice  nbits=24  boolean_output=off  mode=Upper Bit Location + Width  bit1=0  base1=MSB of Input  bit0=24  base0=LSB of Input  dbl_ovrd=off  block_type=slice
  apbw_re_slice3 : xbsIndex_r4/Slice  nbits=24  boolean_output=off  mode=Lower Bit Location + Width  bit1=0  base1=MSB of Input  bit0=0  base0=LSB of Input  dbl_ovrd=off  block_type=slice
  b1 : xbsIndex_r4/Slice  nbits=18  boolean_output=off  mode=Lower Bit Location + Width  bit1=0  base1=MSB of Input  bit0=0  base0=LSB of Input  dbl_ovrd=off  block_type=slice
  b5 : xbsIndex_r4/Slice  nbits=18  boolean_output=off  mode=Lower Bit Location + Width  bit1=0  base1=MSB of Input  bit0=0  base0=LSB of Input  dbl_ovrd=off  block_type=slice
  carryin4 : xbsIndex_r4/Constant  arith_type=Unsigned  const=0  n_bits=1  bin_pt=0  explicit_period=on  period=1  equ=P=C  opselect=C  inp2=PCIN>>17  opr=+  inp1=P  carry=CIN  dbl_ovrd=off  block_type=constant
  carryin8 : xbsIndex_r4/Constant  arith_type=Unsigned  const=0  n_bits=1  bin_pt=0  explicit_period=on  period=1  equ=P=C  opselect=C  inp2=PCIN>>17  opr=+  inp1=P  carry=CIN  dbl_ovrd=off  block_type=constant
  carryinsel4 : xbsIndex_r4/Constant  arith_type=Unsigned  const=0  n_bits=3  bin_pt=0  explicit_period=on  period=1  equ=P=C  opselect=C  inp2=PCIN>>17  opr=+  inp1=P  carry=CIN  dbl_ovrd=off  block_type=constant
  carryinsel8 : xbsIndex_r4/Constant  arith_type=Unsigned  const=0  n_bits=3  bin_pt=0  explicit_period=on  period=1  equ=P=C  opselect=C  inp2=PCIN>>17  opr=+  inp1=P  carry=CIN  dbl_ovrd=off  block_type=constant
  opcode4 : xbsIndex_r4/Constant  arith_type=Unsigned  const=51  n_bits=7  bin_pt=0  explicit_period=on  period=1  equ=P=C  opselect=C  inp2=PCIN>>17  opr=+  inp1=P  carry=CIN  dbl_ovrd=off  block_type=constant
  opcode8 : xbsIndex_r4/Constant  arith_type=Unsigned  const=15  n_bits=7  bin_pt=0  explicit_period=on  period=1  equ=P=C  opselect=C  inp2=PCIN>>17  opr=+  inp1=P  carry=CIN  dbl_ovrd=off  block_type=constant
  a+bw_re : Outport
  a+bw_im : Outport  Port=2
  a-bw_re : Outport  Port=3
  a-bw_im : Outport  Port=4
  wires:
  Concat1/1 -> b1/1, a1/1, Reinterpret1/1
  Concat/1 -> b5/1, a5/1, Reinterpret12/1
  apbw/1 -> apbw_re_slice1/1, apbw_re_slice/1
  ambw/1 -> apbw_re_slice3/1, apbw_re_slice2/1
  opcode8/1 -> apbw/4
  opcode4/1 -> ambw/4
  carryinsel8/1 -> apbw/7
  carryinsel4/1 -> ambw/7
  carryin8/1 -> apbw/6
  carryin4/1 -> ambw/6
  b5/1 -> Reinterpret25/1
  b1/1 -> Reinterpret16/1
  apbw_re_slice3/1 -> Reinterpret4/1
  apbw_re_slice2/1 -> Reinterpret3/1
  apbw_re_slice1/1 -> Reinterpret10/1
  apbw_re_slice/1 -> Reinterpret2/1
  alucode8/1 -> apbw/5
  Reinterpret1/1 -> apbw/3
  Reinterpret25/1 -> apbw/2
  Reinterpret24/1 -> apbw/1
  alucode4/1 -> ambw/5
  Reinterpret12/1 -> ambw/3
  Reinterpret16/1 -> ambw/2
  Reinterpret15/1 -> ambw/1
  a5/1 -> Reinterpret24/1
  a1/1 -> Reinterpret15/1
  Reinterpret8/1 -> Concat1/2
  Convert3/1 -> Reinterpret8/1
  Reinterpret7/1 -> Concat1/1
  Convert2/1 -> Reinterpret7/1
  Reinterpret6/1 -> Concat/2
  Convert1/1 -> Reinterpret6/1
  Reinterpret5/1 -> Concat/1
  Convert/1 -> Reinterpret5/1
  Reinterpret4/1 -> a-bw_im/1
  Reinterpret3/1 -> a-bw_re/1
  Reinterpret2/1 -> a+bw_im/1
  Reinterpret10/1 -> a+bw_re/1
  bw_im/1 -> Convert3/1
  bw_re/1 -> Convert2/1
  a_im/1 -> Convert1/1
  a_re/1 -> Convert/1

== system biplex_unscr_tail_plan/unscr_tail/complex_addsub1/uncram ==
  in : Inport
  Reinterpret15 : xbsIndex_r4/Reinterpret  force_arith_type=on  arith_type="Signed  (2's comp)"  force_bin_pt=on  bin_pt=input_bit_width-1  block_type=reinterpret
      settings: infoedit="Changes signal type without altering the binary representation.   You can changed the signal between signed and unsigned, and relocate the binary point.<br><br>Hardware notes: In hardware this block costs nothing.<br><br>Example:  Suppose the input is 6 bits wide, signed, with 2 fractional bits, and the output is forced to unsigned with 0 fractional bits.  Then an input of -2.0 (1110.00 in binary 2's complement) becomes an output of 56 (111000 in binary)."
  Reinterpret16 : xbsIndex_r4/Reinterpret  force_arith_type=on  arith_type="Signed  (2's comp)"  force_bin_pt=on  bin_pt=input_bit_width-1  block_type=reinterpret
      settings: infoedit="Changes signal type without altering the binary representation.   You can changed the signal between signed and unsigned, and relocate the binary point.<br><br>Hardware notes: In hardware this block costs nothing.<br><br>Example:  Suppose the input is 6 bits wide, signed, with 2 fractional bits, and the output is forced to unsigned with 0 fractional bits.  Then an input of -2.0 (1110.00 in binary 2's complement) becomes an output of 56 (111000 in binary)."
  Slice16 : xbsIndex_r4/Slice  nbits=input_bit_width  boolean_output=off  mode=Upper Bit Location + Width  bit1=-0  base1=MSB of Input  bit0=0  base0=MSB of Input  dbl_ovrd=off  block_type=slice
  Slice17 : xbsIndex_r4/Slice  nbits=input_bit_width  boolean_output=off  mode=Upper Bit Location + Width  bit1=-1* input_bit_width  base1=MSB of Input  bit0=0  base0=MSB of Input  dbl_ovrd=off  block_type=slice
  out0 : Outport
  out1 : Outport  Port=2
  wires:
  Slice16/1 -> Reinterpret15/1
  Reinterpret15/1 -> out0/1
  Slice17/1 -> Reinterpret16/1
  Reinterpret16/1 -> out1/1
  in/1 -> Slice16/1, Slice17/1

== system biplex_unscr_tail_plan/unscr_tail/complex_addsub1/uncram2 ==
  in : Inport
  Reinterpret15 : xbsIndex_r4/Reinterpret  force_arith_type=on  arith_type="Signed  (2's comp)"  force_bin_pt=on  bin_pt=input_bit_width-1  block_type=reinterpret
      settings: infoedit="Changes signal type without altering the binary representation.   You can changed the signal between signed and unsigned, and relocate the binary point.<br><br>Hardware notes: In hardware this block costs nothing.<br><br>Example:  Suppose the input is 6 bits wide, signed, with 2 fractional bits, and the output is forced to unsigned with 0 fractional bits.  Then an input of -2.0 (1110.00 in binary 2's complement) becomes an output of 56 (111000 in binary)."
  Reinterpret16 : xbsIndex_r4/Reinterpret  force_arith_type=on  arith_type="Signed  (2's comp)"  force_bin_pt=on  bin_pt=input_bit_width-1  block_type=reinterpret
      settings: infoedit="Changes signal type without altering the binary representation.   You can changed the signal between signed and unsigned, and relocate the binary point.<br><br>Hardware notes: In hardware this block costs nothing.<br><br>Example:  Suppose the input is 6 bits wide, signed, with 2 fractional bits, and the output is forced to unsigned with 0 fractional bits.  Then an input of -2.0 (1110.00 in binary 2's complement) becomes an output of 56 (111000 in binary)."
  Slice16 : xbsIndex_r4/Slice  nbits=input_bit_width  boolean_output=off  mode=Upper Bit Location + Width  bit1=-0  base1=MSB of Input  bit0=0  base0=MSB of Input  dbl_ovrd=off  block_type=slice
  Slice17 : xbsIndex_r4/Slice  nbits=input_bit_width  boolean_output=off  mode=Upper Bit Location + Width  bit1=-1* input_bit_width  base1=MSB of Input  bit0=0  base0=MSB of Input  dbl_ovrd=off  block_type=slice
  out0 : Outport
  out1 : Outport  Port=2
  wires:
  in/1 -> Slice17/1, Slice16/1
  Reinterpret16/1 -> out1/1
  Slice17/1 -> Reinterpret16/1
  Reinterpret15/1 -> out0/1
  Slice16/1 -> Reinterpret15/1

== system biplex_unscr_tail_plan/unscr_tail/mirror_spectrum/cram1 ==
  in0 : Inport
  in1 : Inport  Port=2
  Concat5 : xbsIndex_r4/Concat  num_inputs=2  dbl_ovrd=off  block_type=concat
  Reinterpret23 : xbsIndex_r4/Reinterpret  force_arith_type=on  arith_type=Unsigned  force_bin_pt=on  bin_pt=0  block_type=reinterpret
      settings: infoedit="Changes signal type without altering the binary representation.   You can changed the signal between signed and unsigned, and relocate the binary point.<br><br>Hardware notes: In hardware this block costs nothing.<br><br>Example:  Suppose the input is 6 bits wide, signed, with 2 fractional bits, and the output is forced to unsigned with 0 fractional bits.  Then an input of -2.0 (1110.00 in binary 2's complement) becomes an output of 56 (111000 in binary)."
  Reinterpret24 : xbsIndex_r4/Reinterpret  force_arith_type=on  arith_type=Unsigned  force_bin_pt=on  bin_pt=0  block_type=reinterpret
      settings: infoedit="Changes signal type without altering the binary representation.   You can changed the signal between signed and unsigned, and relocate the binary point.<br><br>Hardware notes: In hardware this block costs nothing.<br><br>Example:  Suppose the input is 6 bits wide, signed, with 2 fractional bits, and the output is forced to unsigned with 0 fractional bits.  Then an input of -2.0 (1110.00 in binary 2's complement) becomes an output of 56 (111000 in binary)."
  out : Outport
  wires:
  Concat5/1 -> out/1
  in0/1 -> Reinterpret23/1
  Reinterpret23/1 -> Concat5/1
  in1/1 -> Reinterpret24/1
  Reinterpret24/1 -> Concat5/2

== system biplex_unscr_tail_plan/unscr_tail/mirror_spectrum/cram2 ==
  in0 : Inport
  in1 : Inport  Port=2
  Concat6 : xbsIndex_r4/Concat  num_inputs=2  dbl_ovrd=off  block_type=concat
  Reinterpret25 : xbsIndex_r4/Reinterpret  force_arith_type=on  arith_type=Unsigned  force_bin_pt=on  bin_pt=0  block_type=reinterpret
      settings: infoedit="Changes signal type without altering the binary representation.   You can changed the signal between signed and unsigned, and relocate the binary point.<br><br>Hardware notes: In hardware this block costs nothing.<br><br>Example:  Suppose the input is 6 bits wide, signed, with 2 fractional bits, and the output is forced to unsigned with 0 fractional bits.  Then an input of -2.0 (1110.00 in binary 2's complement) becomes an output of 56 (111000 in binary)."
  Reinterpret26 : xbsIndex_r4/Reinterpret  force_arith_type=on  arith_type=Unsigned  force_bin_pt=on  bin_pt=0  block_type=reinterpret
      settings: infoedit="Changes signal type without altering the binary representation.   You can changed the signal between signed and unsigned, and relocate the binary point.<br><br>Hardware notes: In hardware this block costs nothing.<br><br>Example:  Suppose the input is 6 bits wide, signed, with 2 fractional bits, and the output is forced to unsigned with 0 fractional bits.  Then an input of -2.0 (1110.00 in binary 2's complement) becomes an output of 56 (111000 in binary)."
  out : Outport
  wires:
  Concat6/1 -> out/1
  in0/1 -> Reinterpret25/1
  Reinterpret25/1 -> Concat6/1
  in1/1 -> Reinterpret26/1
  Reinterpret26/1 -> Concat6/2

== system biplex_unscr_tail_plan/unscr_tail/mirror_spectrum/cram3 ==
  in0 : Inport
  in1 : Inport  Port=2
  Concat7 : xbsIndex_r4/Concat  num_inputs=2  dbl_ovrd=off  block_type=concat
  Reinterpret27 : xbsIndex_r4/Reinterpret  force_arith_type=on  arith_type=Unsigned  force_bin_pt=on  bin_pt=0  block_type=reinterpret
      settings: infoedit="Changes signal type without altering the binary representation.   You can changed the signal between signed and unsigned, and relocate the binary point.<br><br>Hardware notes: In hardware this block costs nothing.<br><br>Example:  Suppose the input is 6 bits wide, signed, with 2 fractional bits, and the output is forced to unsigned with 0 fractional bits.  Then an input of -2.0 (1110.00 in binary 2's complement) becomes an output of 56 (111000 in binary)."
  Reinterpret28 : xbsIndex_r4/Reinterpret  force_arith_type=on  arith_type=Unsigned  force_bin_pt=on  bin_pt=0  block_type=reinterpret
      settings: infoedit="Changes signal type without altering the binary representation.   You can changed the signal between signed and unsigned, and relocate the binary point.<br><br>Hardware notes: In hardware this block costs nothing.<br><br>Example:  Suppose the input is 6 bits wide, signed, with 2 fractional bits, and the output is forced to unsigned with 0 fractional bits.  Then an input of -2.0 (1110.00 in binary 2's complement) becomes an output of 56 (111000 in binary)."
  out : Outport
  wires:
  Concat7/1 -> out/1
  in0/1 -> Reinterpret27/1
  Reinterpret27/1 -> Concat7/1
  in1/1 -> Reinterpret28/1
  Reinterpret28/1 -> Concat7/2
